simulink model "sampling_tf"  (R2018b)
settings: Solver=VariableStepAuto  StartTime=0.0  StopTime=39  RelTol=1e-3
settings Model: Creator=Fangming  LastModifiedBy=iamcy

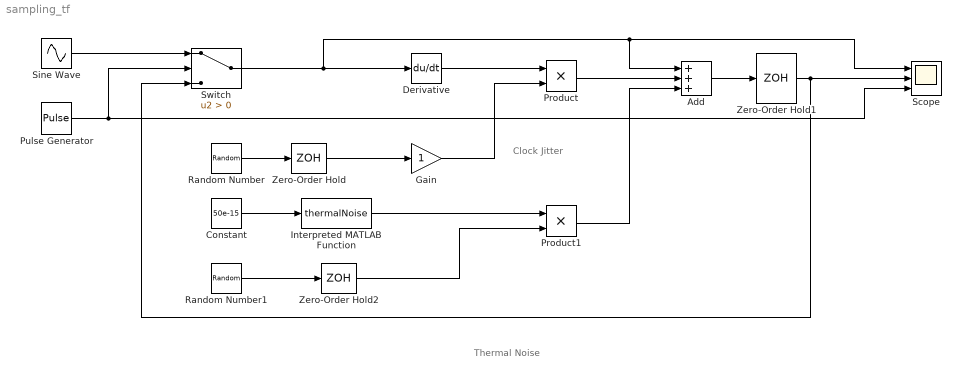
== system sampling_tf ==
  note: Clock Jitter
  note: Thermal Noise
  Add : Sum  Inputs=3
  Constant : Constant  Value=50e-15
  Derivative : Derivative  CoefficientInTFapproximation=0
  Gain : Gain
  Interpreted MATLAB Function : MATLABFcn  MATLABFcn=thermalNoise
  Product : Product
  Product1 : Product
  Pulse Generator : DiscretePulseGenerator  PulseType=Time based  Period=13  PulseWidth=100/13
  Random Number : RandomNumber  Variance=30e-12  SampleTime=0.1
  Random Number1 : RandomNumber  Variance=30e-12  SampleTime=0.1
  Scope : Scope  NumInputPorts=3
  Sine Wave : Sin  Frequency=0.01  SampleTime=0
  Switch : Switch  Criteria=u2 > Threshold
  Zero-Order Hold : ZeroOrderHold  SampleTime=-1
  Zero-Order Hold1 : ZeroOrderHold  SampleTime=13
  Zero-Order Hold2 : ZeroOrderHold  SampleTime=-1
  wires:
  Random Number/1 -> Zero-Order Hold/1
  Gain/1 -> Product/2
  Derivative/1 -> Product/1
  Product/1 -> Add/2
  Sine Wave/1 -> Switch/1
  Pulse Generator/1 -> Switch/2, Scope/3
  Zero-Order Hold/1 -> Gain/1
  Switch/1 -> Scope/1, Add/1, Derivative/1
  Add/1 -> Zero-Order Hold1/1
  Zero-Order Hold1/1 -> Switch/3, Scope/2
  Constant/1 -> Interpreted MATLAB Function/1
  Interpreted MATLAB Function/1 -> Product1/1
  Random Number1/1 -> Zero-Order Hold2/1
  Zero-Order Hold2/1 -> Product1/2
  Product1/1 -> Add/3
